simulink model "AddMemoria"  (R2022a)
settings: Solver=VariableStepAuto  StartTime=0.0  StopTime=10.0  RelTol=1e-3
settings Model: Creator=Usuario  LastModifiedBy=Usuario

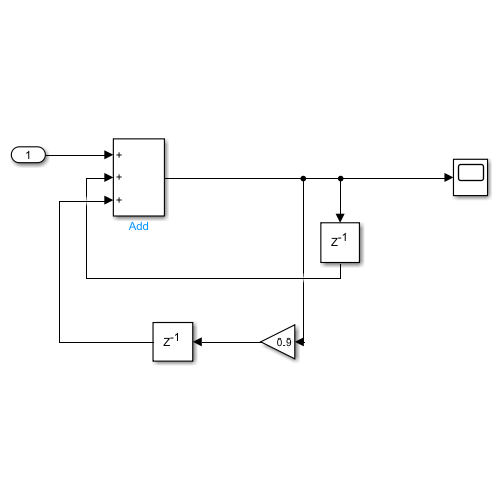
[thumbnail: Simulink's stored preview of the top-level diagram]
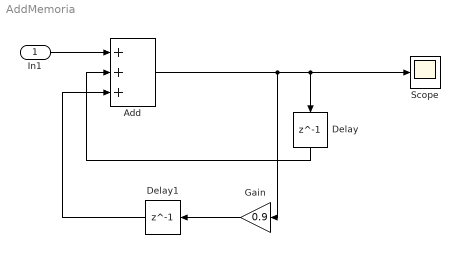
== system AddMemoria ==
  In1 : Inport
  Add : Sum  Inputs=+++
  Delay : Delay  DelayLength=1  InitialCondition=0
  Delay1 : Delay  DelayLength=1  InitialCondition=0
  Gain : Gain  Gain=0.9
  Scope : Scope
  wires:
  In1/1 -> Add/1
  Add/1 -> Delay/1, Scope/1, Gain/1
  Delay/1 -> Add/2
  Gain/1 -> Delay1/1
  Delay1/1 -> Add/3
